simulink model "UNICO"  (R2023b)
settings: Solver=FixedStepDiscrete  StartTime=0.0  StopTime=inf  FixedStep=Control.DT  RelTol=1e-3
values from neighbouring files (symbols this model uses):
  Control =     [Parameters_UNICO.mat]
libraries: simulink x2
(part 1 of 3)
settings Model: Creator=evansolingen  LastModifiedBy=STUDENTE
settings SolverCC: AlgebraicLoopSolver=TrustRegion
settings DataIOCC: LimitDataPoints=on  SaveFormat=Array  SignalLoggingSaveFormat=ModelDataLogs  SaveOutput=off  SignalLogging=off  SaveTime=off  ReturnWorkspaceOutputs=off
settings OptimizationCC: BlockReduction=off  DefaultParameterBehavior=Inlined  BufferReuse=off  ReuseModelBlockBuffer=off  ExpressionDepthLimit=2147483647  LifeSpan=inf
settings DebuggingCC: UnderspecifiedInitializationDetection=Classic  MergeDetectMultiDrivingBlocksExec=none  SolverPrmCheckMsg=warning  MultiTaskDSMMsg=warning  MultiTaskCondExecSysMsg=none  FcnCallInpInsideContextMsg=warning  UnconnectedInputMsg=warning  UnconnectedOutputMsg=warning  UnconnectedLineMsg=warning  AllowSymbolicDim=off  StateNameClashWarn=warning  SFUnexpectedBacktrackingDiag=warning  SFNoUnconditionalDefaultTransitionDiag=warning  SFExecutionAtInitializationDiag=none  ArithmeticOperatorsInVariantConditions=warning
settings HardwareCC: ProdBitPerPointer=32  ProdBitPerSizeT=32  ProdBitPerPtrDiffT=32  ProdLargestAtomicFloat=None  ProdIntDivRoundTo=Undefined  ProdEndianess=Unspecified  ProdWordSize=32  ProdHWDeviceType=32-bit Generic
settings ModelReferenceCC: UpdateModelReferenceTargets=Force  EnableRefExpFcnMdlSchedulingChecks=on  PropagateSignalLabelsOutOfModel=off
settings SFSimCC: SimUseLocalCustomCode=off  SimParseCustomCode=off  CustomCodeUndefinedFunction=UseInterfaceOnly
settings RTWCC: Description=DISCON DLL Target (for use with GH BLADED)  SystemTargetFile=discon.tlc  TemplateMakefile=discon_vc.tmf  RTWUseLocalCustomCode=off
settings CodeAppCC: StateflowObjectComments=on
settings GRTTargetCC: TargetLangStandard=C89/C90 (ANSI)  CombineOutputUpdateFcns=off  GRTInterface=on  UseToolchainInfoCompliant=off  ExtModeMexFile=noextcomm
settings ConfigComp: CovMetricSettings=dw  CovSaveCumulativeToWorkspaceVar=on  CovSaveSingleToWorkspaceVar=on  CovExternalEMLEnable=off

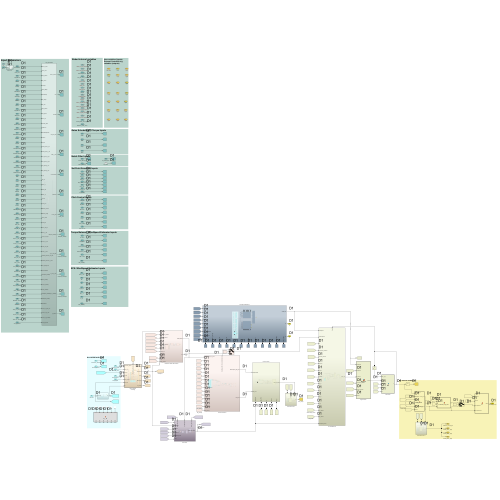
[thumbnail: Simulink's stored preview of the top-level diagram]
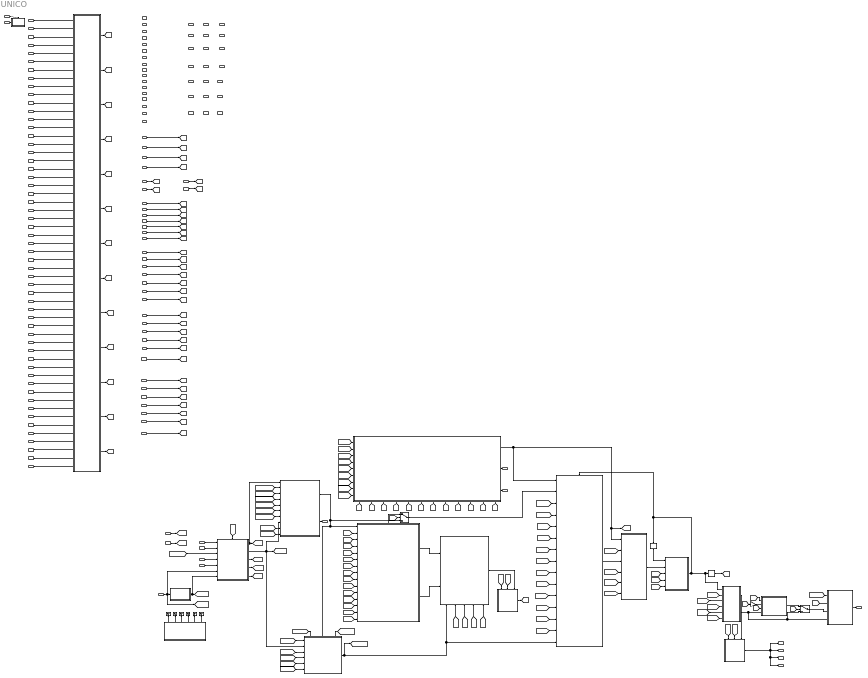
== system UNICO ==
  note: Bladed internal variables
  note: User variables (inputs)
      | External Controller log variables (outputs)
  note: Input parameters
  note: DLL OUTPUT INTERFACE
  note: DLL INTERFACE inputs
  note: Gains Scheduling PI Torque Inputs
  note: Torque Balance - WindSpeed Estimator Inputs
  note: Set Point Smoother Inputs
  note: EFK- WindSpeed Estimator Inputs
  note: Notch Filter Inputs
  note: Pitch Control Inputs
  Rated_Speed : Inport  PortDimensions=1
  Mode_Gain : Inport  Port=2  PortDimensions=1
  Blade1_OP_Root_Moment : Inport  Port=3  PortDimensions=1
  Blade2_OP_Root_Moment : Inport  Port=4  PortDimensions=1
  Blade3_OP_Root_Moment : Inport  Port=5  PortDimensions=1
  Rotor_Azimuth_Angle : Inport  Port=6  PortDimensions=1
  Init : Inport  Port=7  PortDimensions=1
  Shaft_Torque : Inport  Port=8  PortDimensions=1
  Blade1_IP_Root_Moment : Inport  Port=9  PortDimensions=1
  Blade2_IP_Root_Moment : Inport  Port=10  PortDimensions=1
  Blade3_IP_Root_Moment : Inport  Port=11  PortDimensions=1
  YawError : Inport  Port=12  PortDimensions=1
  YawBearingRate : Inport  Port=13  PortDimensions=1
  ElectricalPower : Inport  Port=14  PortDimensions=1
  Fore_Aft_Tower_Accel : Inport  Port=15  PortDimensions=1
  Generator_Speed : Inport  Port=16  PortDimensions=1
  Sidewards_Tower_Accel : Inport  Port=17  PortDimensions=1
  Below_Rated_Pitch_Angle : Inport  Port=18  PortDimensions=1
  Wind_Speed : Inport  Port=19  PortDimensions=1
  Com_dt : Inport  Port=20  PortDimensions=1
  SimTime : Inport  Port=21
  dKSwitch : Inport  Port=22  SampleTime=Control.DT  Interpolate=off  LockScale=on
  dRgn2K : Inport  Port=23  PortDimensions=1
  dOMSpdSwitch : Inport  Port=24  PortDimensions=1
  dRotorRadius : Inport  Port=25  PortDimensions=1
  dRgn3Mode : Inport  Port=26  PortDimensions=1
  dMRgn3Lin : Inport  Port=27  PortDimensions=1
  dGenEff : Inport  Port=28  PortDimensions=1
  dMinOMSpd : Inport  Port=29  PortDimensions=1
  dRtWSpd : Inport  Port=30  PortDimensions=1
  dRhoAir : Inport  Port=31  PortDimensions=1
  dRtPwr : Inport  Port=32  PortDimensions=1
  dRtGenSpd : Inport  Port=33  PortDimensions=1
  dTSRopt : Inport  Port=34  PortDimensions=1
  dRgn2Mode : Inport  Port=35  PortDimensions=1
  dWindSpeedFSw : Inport  Port=36
  dWindSpeedFLPF : Inport  Port=37
  dGenSpeedFSw : Inport  Port=38
  dGenSpeedFLPF : Inport  Port=39
  dRefSpeedFSw : Inport  Port=40
  dRefSpeedFLPF : Inport  Port=41
  dVLin : Inport  Port=42
  dMaxRat : Inport  Port=43  PortDimensions=1
  dMaxTq : Inport  Port=44  PortDimensions=1
  dMinTq : Inport  Port=45  PortDimensions=1
  dRtTq : Inport  Port=46  PortDimensions=1
  dEcho : Inport  Port=47
  dCpMax : Inport  Port=48
  dFPitch : Inport  Port=49
  Measured_Torque : Inport  Port=50
  dMinOMSpdSwitch : Inport  Port=51  PortDimensions=1
  Architecture_Selector : Inport  Port=52
  dZeros_Damping : Inport  Port=53
  dPoles_Damping : Inport  Port=54
  dBlades_Number : Inport  Port=55
  dBlades_Height : Inport  Port=56
  dAWSwitch : Inport  Port=57
  dKpBr : Inport  Port=58  PortDimensions=1
  dRotInertia : Inport  Port=59
  dIntTermSwitch : Inport  Port=60
  dKiBr : Inport  Port=61  PortDimensions=1
  dKpAr : Inport  Port=62  PortDimensions=1
  dKiAr : Inport  Port=63  PortDimensions=1
  dTSR_R3 : Inport  Port=64
  Measured_Pitch : Inport  Port=65  PortDimensions=1
  Pitch_LPF_Sw : Inport  Port=66
  Torque_in_LPF_Sw : Inport  Port=67
  Power_LPF_Sw : Inport  Port=68
  Pitch_F_LPF : Inport  Port=69
  Torque_in_F_LPF : Inport  Port=70
  Power_F_LPF : Inport  Port=71
  SPS_LPF_Sw : Inport  Port=72
  SPS_F_LPF : Inport  Port=73
  SPS_Mode : Inport  Port=74
  SPS_Kvs : Inport  Port=75
  SPS_Kpc : Inport  Port=76
  SPS_Abbas_Factor : Inport  Port=77
  Max_Pitch : Inport  Port=78
  Pitch_Rate : Inport  Port=79
  LPF_StartingTime : Inport  Port=80
  WSE_Mode : Inport  Port=81
  GearBox_Ratio : Inport  Port=82
  Darrieus_Selector : Inport  Port=83
  Rotor_Area : Inport  Port=84
  Process_Noise_Q : Inport  Port=85
  Measurement_Noise_R : Inport  Port=86
  TBE_F_LPF : Inport  Port=87
  EKF_F_LPF : Inport  Port=88
  Rm : Inport  Port=89
  Ti : Inport  Port=90
  PS_LPF_Sw : Inport  Port=91
  PS_F_LPF : Inport  Port=92
  Min_Pitch : Inport  Port=93
  PC_Kp : Inport  Port=94
  PC_Ki : Inport  Port=95
  Cp_interp : Inport  Port=96
  Cp_opt_in : Inport  Port=97
  Cp_2_in : Inport  Port=98
  A_op : Inport  Port=99
  WindSpeed_PreWarp : Inport  Port=100
  GenSpeed_PreWarp : Inport  Port=101
  RefSpeed_PreWarp : Inport  Port=102
  Pitch_PreWarp : Inport  Port=103
  Torque_in_PreWarp : Inport  Port=104
  TBE_PreWarp : Inport  Port=105
  EKF_PreWarp : Inport  Port=106
  Power_PreWarp : Inport  Port=107
  SPS_PreWarp : Inport  Port=108
  PS_PreWarp : Inport  Port=109
  Pitch_Ctrl_Sw : Inport  Port=110
  Torque_out_LPF_Sw : Inport  Port=111
  Torque_out_F_LPF : Inport  Port=112
  Torque_out_PreWarp : Inport  Port=113
  NF_StartingTime : Inport  Port=114
  NF_Switch : Inport  Port=115
  omega_stallmin : Inport  Port=116
  Delay One Step : Delay  DelayLength=1
  Delay One Step3 : Delay  DelayLength=1
  Echo print : Subsystem
      settings: PortSchema="{\"entries\":[{\"content\":{\"sides\":[{\"content\":{\"connectorIds\":[\"In1\"]},\"type\":\"ConnectorPlacement.EquallySpacedRectSide\",\"uuid\":\"a7404841-4279-4901-8e4b-4d9f651fd70d\"},{\"content\":{\"side\":\"RIGHT\"},\"type\":\"ConnectorPlacement.EquallySpacedRectSide\",\"uuid\":\"c083252d-994d-448b-85dd-b05fa098362a\"},{\"content\":{\"connectorIds\":[\"In2\"],\"side\":\"TOP\"},\"type\":\"ConnectorPlacement.EquallySpacedRectSide\",\"uuid\":\"2158789e-5709-45dd-87ec-c3c83921db3a\"}]},\"type\":\"ConnectorPlacement.EquallySpacedConnector\",\"uuid\":\"2f3f8f4d-3210-4d41-988d-02cc8661526f\"}],\"packageUris\":[\"http://schema.mathworks.com/mf0/Connector/R2020b\"],\"version\":\"1.0\"}"
  Extract Signals & Filtering : Subsystem  TreatAsAtomicUnit=on
      settings: PortSchema="{\"entries\":[{\"content\":{\"sides\":[{\"content\":{\"connectorIds\":[\"In1\",\"In2\",\"In3\",\"In4\",\"In5\",\"In6\",\"In7\"]},\"type\":\"ConnectorPlacement.EquallySpacedRectSide\",\"uuid\":\"a404705e-4872-4bcb-ba41-9c444b954adf\"},{\"content\":{\"connectorIds\":[\"Out1\",\"Out2\",\"Out3\",\"Out4\",\"Out5\"],\"side\":\"RIGHT\"},\"type\":\"ConnectorPlacement.EquallySpacedRectSide\",\"uuid\":\"c545baa2-32cf-46ec-85e6-24376232facc\"},{\"content\":{\"connectorIds\":[\"In8\"],\"side\":\"TOP\"},\"type\":\"ConnectorPlacement.EquallySpacedRectSide\",\"uuid\":\"109e9702-ec3d-43ff-9af6-4bdbb05ed40a\"}]},\"type\":\"ConnectorPlacement.EquallySpacedConnector\",\"uuid\":\"3e4fa54c-da00-45a5-8912-ad9d54069fc2\"}],\"packageUris\":[\"http://schema.mathworks.com/mf0/Connector/R2020b\"],\"version\":\"1.0\"}"
  Gain4 : Gain  Gain=2*pi
  Input_parameters : Subsystem
  MATLAB Function1 : MATLAB Function  TreatAsAtomicUnit=on
  MATLAB Function2 : MATLAB Function  TreatAsAtomicUnit=on
  MATLAB Function3 : MATLAB Function  TreatAsAtomicUnit=on
  MATLAB Function4 : MATLAB Function  TreatAsAtomicUnit=on
  Notch Filter : Subsystem
      settings: PortSchema="{\"entries\":[{\"content\":{\"sides\":[{\"content\":{\"connectorIds\":[\"In1\",\"In2\",\"In3\",\"In4\",\"In5\",\"In6\"]},\"type\":\"ConnectorPlacement.EquallySpacedRectSide\",\"uuid\":\"266d7f1f-a9f2-4128-b770-569d38332992\"},{\"content\":{\"connectorIds\":[\"Out1\"],\"side\":\"RIGHT\"},\"type\":\"ConnectorPlacement.EquallySpacedRectSide\",\"uuid\":\"006e736b-d915-4b42-8363-b4fafec53ea5\"},{\"content\":{\"connectorIds\":[\"In7\",\"In8\",\"In9\"],\"side\":\"TOP\"},\"type\":\"ConnectorPlacement.EquallySpacedRectSide\",\"uuid\":\"979f8782-bd32-4411-8fc6-7070b3b90e64\"},{\"content\":{\"side\":\"BOTTOM\"},\"type\":\"ConnectorPlacement.EquallySpacedRectSide\",\"uuid\":\"d10cf628-97fc-4eef-9b08-34d81c8bbc38\"}]},\"type\":\"ConnectorPlacement.EquallySpacedConnector\",\"uuid\":\"1a915c26-6e95-4b6d-8a27-3bc1b56b8115\"}],\"packageUris\":[\"http://schema.mathworks.com/mf0/Connector/R2020b\"],\"version\":\"1.0\"}"
  PI CONTROLLER : Subsystem
      settings: PortSchema="{\"entries\":[{\"content\":{\"sides\":[{\"content\":{\"connectorIds\":[\"In1\",\"In2\",\"In3\",\"In4\",\"In5\",\"In6\",\"In7\",\"In8\",\"In9\",\"In10\",\"In11\",\"In12\",\"In13\",\"In14\",\"In15\"]},\"type\":\"ConnectorPlacement.EquallySpacedRectSide\",\"uuid\":\"cac6f54d-e2c8-43c6-b064-9a31ea99ed9a\"},{\"content\":{\"connectorIds\":[\"Out1\"],\"side\":\"RIGHT\"},\"type\":\"ConnectorPlacement.EquallySpacedRectSide\",\"uuid\":\"e149802a-12fb-4560-9018-b92a983da9c3\"},{\"content\":{\"connectorIds\":[\"In16\"],\"side\":\"TOP\"},\"type\":\"ConnectorPlacement.EquallySpacedRectSide\",\"uuid\":\"c9e2d139-52ab-4592-996b-9b011a50426a\"}]},\"type\":\"ConnectorPlacement.EquallySpacedConnector\",\"uuid\":\"845cf794-e810-4ec5-9bce-289872a07b1e\"}],\"packageUris\":[\"http://schema.mathworks.com/mf0/Connector/R2020b\"],\"version\":\"1.0\"}"
  Pitch Controller : Subsystem
      settings: PortSchema="{\"entries\":[{\"content\":{\"sides\":[{\"content\":{\"connectorIds\":[\"In1\",\"In2\"]},\"type\":\"ConnectorPlacement.EquallySpacedRectSide\",\"uuid\":\"15f3ef00-8fd2-4b01-b950-6d151530d8d8\"},{\"content\":{\"connectorIds\":[\"Out1\"],\"side\":\"RIGHT\"},\"type\":\"ConnectorPlacement.EquallySpacedRectSide\",\"uuid\":\"9a379538-e873-4d9a-b3d5-9d5b8b382616\"},{\"content\":{\"side\":\"TOP\"},\"type\":\"ConnectorPlacement.EquallySpacedRectSide\",\"uuid\":\"382e266d-b53f-4a4d-a6cd-b7a4030212ef\"},{\"content\":{\"connectorIds\":[\"In3\",\"In4\",\"In5\",\"In6\",\"In7\"],\"side\":\"BOTTOM\"},\"type\":\"ConnectorPlacement.EquallySpacedRectSide\",\"uuid\":\"ee17fbc2-2aec-488d-9e0d-2e4dec5ded05\"}]},\"type\":\"ConnectorPlacement.EquallySpacedConnector\",\"uuid\":\"dba4a2db-8eaa-452b-8e55-416d9caf5878\"}],\"packageUris\":[\"http://schema.mathworks.com/mf0/Connector/R2020b\"],\"version\":\"1.0\"}"
  Pitch Rate Limiter : Subsystem
      settings: PortSchema="{\"entries\":[{\"content\":{\"sides\":[{\"content\":{\"connectorIds\":[\"In1\",\"In2\",\"In3\"]},\"type\":\"ConnectorPlacement.EquallySpacedRectSide\",\"uuid\":\"71de1963-385a-424e-a4e7-bb08b9d03775\"},{\"content\":{\"side\":\"RIGHT\"},\"type\":\"ConnectorPlacement.EquallySpacedRectSide\",\"uuid\":\"e3763a80-b3da-4c7c-ac2e-798dc78d2a39\"},{\"content\":{\"side\":\"TOP\"},\"type\":\"ConnectorPlacement.EquallySpacedRectSide\",\"uuid\":\"c338073c-3d17-477d-80b8-b5d5ee58aec7\"},{\"content\":{\"connectorIds\":[\"Out1\"],\"side\":\"BOTTOM\"},\"type\":\"ConnectorPlacement.EquallySpacedRectSide\",\"uuid\":\"70822ac6-7ea9-4832-9fee-c86b7b7e7f31\"}]},\"type\":\"ConnectorPlacement.EquallySpacedConnector\",\"uuid\":\"46c33881-c4d8-4782-931d-07fcd796c079\"}],\"packageUris\":[\"http://schema.mathworks.com/mf0/Connector/R2020b\"],\"version\":\"1.0\"}"
  Pitch Rate Limiter1 : Subsystem
      settings: PortSchema="{\"entries\":[{\"content\":{\"sides\":[{\"content\":{\"connectorIds\":[\"In1\",\"In2\",\"In3\"]},\"type\":\"ConnectorPlacement.EquallySpacedRectSide\",\"uuid\":\"71de1963-385a-424e-a4e7-bb08b9d03775\"},{\"content\":{\"side\":\"RIGHT\"},\"type\":\"ConnectorPlacement.EquallySpacedRectSide\",\"uuid\":\"e3763a80-b3da-4c7c-ac2e-798dc78d2a39\"},{\"content\":{\"side\":\"TOP\"},\"type\":\"ConnectorPlacement.EquallySpacedRectSide\",\"uuid\":\"c338073c-3d17-477d-80b8-b5d5ee58aec7\"},{\"content\":{\"connectorIds\":[\"Out1\"],\"side\":\"BOTTOM\"},\"type\":\"ConnectorPlacement.EquallySpacedRectSide\",\"uuid\":\"70822ac6-7ea9-4832-9fee-c86b7b7e7f31\"}]},\"type\":\"ConnectorPlacement.EquallySpacedConnector\",\"uuid\":\"46c33881-c4d8-4782-931d-07fcd796c079\"}],\"packageUris\":[\"http://schema.mathworks.com/mf0/Connector/R2020b\"],\"version\":\"1.0\"}"
  Rate limiter : MATLAB Function  TreatAsAtomicUnit=on
  Reference Speed Determination : Subsystem
  "Region Switch " : MATLAB Function  TreatAsAtomicUnit=on
  Set Point Smoother : Subsystem
      settings: PortSchema="{\"entries\":[{\"content\":{\"sides\":[{\"content\":{\"connectorIds\":[\"In1\",\"In2\",\"In3\",\"In4\",\"In5\",\"In6\",\"In7\",\"In8\",\"In9\",\"In10\",\"In11\",\"In12\",\"In13\",\"In14\",\"In15\"]},\"type\":\"ConnectorPlacement.EquallySpacedRectSide\",\"uuid\":\"b45f5cc4-c36d-4f69-abed-54c577fa7509\"},{\"content\":{\"connectorIds\":[\"Out1\",\"Out2\"],\"side\":\"RIGHT\"},\"type\":\"ConnectorPlacement.EquallySpacedRectSide\",\"uuid\":\"93d4c31e-6d03-43b5-9766-df680cc2625e\"},{\"content\":{\"connectorIds\":[\"Out3\"],\"side\":\"TOP\"},\"type\":\"ConnectorPlacement.EquallySpacedRectSide\",\"uuid\":\"bbab9ad3-67d7-4805-8de6-8e5f911d7e32\"}]},\"type\":\"ConnectorPlacement.EquallySpacedConnector\",\"uuid\":\"cc63daf0-1a6c-427a-a186-92445beec46e\"}],\"packageUris\":[\"http://schema.mathworks.com/mf0/Connector/R2020b\"],\"version\":\"1.0\"}"
  Subsystem1 : Subsystem
  Switch : Switch  Criteria=u2 ~= 0  SaturateOnIntegerOverflow=off  InputSameDT=off
  Switch3 : Switch  Criteria=u2 ~= 0  SaturateOnIntegerOverflow=off  InputSameDT=off
  Terminator{1..6} (6 alike) : Terminator
  Wind Speed Estimators : Subsystem
      settings: PortSchema="{\"entries\":[{\"content\":{\"sides\":[{\"content\":{\"connectorIds\":[\"In1\",\"In2\",\"In3\",\"In4\",\"In5\",\"In6\",\"In7\",\"In8\",\"In9\"]},\"type\":\"ConnectorPlacement.EquallySpacedRectSide\",\"uuid\":\"93f714cb-9c59-4e12-ade1-e7df00512455\"},{\"content\":{\"connectorIds\":[\"Out1\",\"Out2\",\"Out3\"],\"side\":\"RIGHT\"},\"type\":\"ConnectorPlacement.EquallySpacedRectSide\",\"uuid\":\"d5526135-9f63-41d7-93a5-f87b80e4f455\"},{\"content\":{\"side\":\"TOP\"},\"type\":\"ConnectorPlacement.EquallySpacedRectSide\",\"uuid\":\"82fe9337-8013-44e5-aac2-a73e686a79d7\"},{\"content\":{\"connectorIds\":[\"In10\",\"In11\",\"In12\",\"In13\",\"In14\",\"In15\",\"In16\",\"In17\",\"In18\",\"In19\",\"In20\",\"In21\"],\"side\":\"BOTTOM\"},\"type\":\"ConnectorPlacement.EquallySpacedRectSide\",\"uuid\":\"b65e2683-3e9b-43b5-8446-61ba0d8b1898\"}]},\"type\":\"ConnectorPlacement.EquallySpacedConnector\",\"uuid\":\"740892b4-794b-4135-9713-ff5336da8300\"}],\"packageUris\":[\"http://schema.mathworks.com/mf0/Connector/R2020b\"],\"version\":\"1.0\"}"
  Log3 : Outport  PortDimensions=1  VectorParamsAs1DForOutWhenUnconnected=off
  Log4 : Outport  Port=2  PortDimensions=1  VectorParamsAs1DForOutWhenUnconnected=off
  Log5 : Outport  Port=3  PortDimensions=1  VectorParamsAs1DForOutWhenUnconnected=off
  Log6 : Outport  Port=4  PortDimensions=1  VectorParamsAs1DForOutWhenUnconnected=off
  Log7 : Outport  Port=5  PortDimensions=1  VectorParamsAs1DForOutWhenUnconnected=off
  Log10 : Outport  Port=6  PortDimensions=1  VectorParamsAs1DForOutWhenUnconnected=off
  Log8 : Outport  Port=7  PortDimensions=1  VectorParamsAs1DForOutWhenUnconnected=off
  Log20 : Outport  Port=8  PortDimensions=1  VectorParamsAs1DForOutWhenUnconnected=off
  Log12 : Outport  Port=9  PortDimensions=1  VectorParamsAs1DForOutWhenUnconnected=off
  Log17 : Outport  Port=10  PortDimensions=1  VectorParamsAs1DForOutWhenUnconnected=off
  Log18 : Outport  Port=11  PortDimensions=1  VectorParamsAs1DForOutWhenUnconnected=off
  Log19 : Outport  Port=12  PortDimensions=1  VectorParamsAs1DForOutWhenUnconnected=off
  Log13 : Outport  Port=13  PortDimensions=1  VectorParamsAs1DForOutWhenUnconnected=off
  Log14 : Outport  Port=14  PortDimensions=1  VectorParamsAs1DForOutWhenUnconnected=off
  Log15 : Outport  Port=15  PortDimensions=1  VectorParamsAs1DForOutWhenUnconnected=off
  Log1 : Outport  Port=16  PortDimensions=1  VectorParamsAs1DForOutWhenUnconnected=off
  Log16 : Outport  Port=17  PortDimensions=1  VectorParamsAs1DForOutWhenUnconnected=off
  Log2 : Outport  Port=18  PortDimensions=1  VectorParamsAs1DForOutWhenUnconnected=off
  Log9 : Outport  Port=19  PortDimensions=1  VectorParamsAs1DForOutWhenUnconnected=off
  Log11 : Outport  Port=20  PortDimensions=1  VectorParamsAs1DForOutWhenUnconnected=off
  Yaw_Rate : Outport  Port=21  PortDimensions=1  VectorParamsAs1DForOutWhenUnconnected=off
  Blade1_Pitch_Angle : Outport  Port=22  PortDimensions=1  VectorParamsAs1DForOutWhenUnconnected=off
  Blade2_Pitch_Angle : Outport  Port=23  PortDimensions=1  VectorParamsAs1DForOutWhenUnconnected=off
  Blade3_Pitch_Angle : Outport  Port=24  PortDimensions=1  VectorParamsAs1DForOutWhenUnconnected=off
  Collective_Pitch_Angle : Outport  Port=25  PortDimensions=1  VectorParamsAs1DForOutWhenUnconnected=off
  vh : Outport  Port=26
  vw : Outport  Port=27
  Generator_Torque : Outport  Port=28  PortDimensions=1  VectorParamsAs1DForOutWhenUnconnected=off
  Cp : Outport  Port=29
  tag scope: InPar=global, KiAr=global, KiBr=global, KpAr=global, KpBr=global, LPF=global, MaxRat=global, SPS_F_LPF=global, SPS_F_Sw=global
  wires:
  dRhoAir/1 -> Input_parameters/4(dAir_Dens)
  dMaxRat/1 -> Input_parameters/27(dMax_Rat)
  dRgn2K/1 -> Input_parameters/17(Rgn2K)
  Init/1 -> Echo print/1(Init)
  dKSwitch/1 -> Input_parameters/16(KSwitch)
  dFPitch/1 -> Input_parameters/30(fixed_pitch)
  dTSRopt/1 -> Input_parameters/5(dTSRopt)
  Input_parameters/2(LPF) -> [LPF]
  dWindSpeedFLPF/1 -> Input_parameters/19(Wind_Speed_F_LPF)
  dRgn2Mode/1 -> Input_parameters/3(dRgn2_Mode)
  Input_parameters/1(Discon_Params) -> [InPar]
  dEcho/1 -> Echo print/2(Echo)
  dRefSpeedFLPF/1 -> Input_parameters/23(Ref_Speed_F_LPF)
  dRtTq/1 -> Input_parameters/25(dRt_Tq)
  dVLin/1 -> Input_parameters/24(V_lin)
  dRefSpeedFSw/1 -> Input_parameters/22(Ref_Speed_F_Sw)
  dRtGenSpd/1 -> Input_parameters/7(dRatGenSpd)
  dMaxTq/1 -> Input_parameters/28(dMax_Tq)
  dOMSpdSwitch/1 -> Input_parameters/14(SpdSwitch)
  dRgn3Mode/1 -> Input_parameters/10(dRgn3_Mode)
  dCpMax/1 -> Input_parameters/29(Cpmax)
  dRotorRadius/1 -> Input_parameters/1(dRotor_radius)
  dRtWSpd/1 -> Input_parameters/8(dRt_WSpd)
  dMinTq/1 -> Input_parameters/26(dMin_Tq)
  dMinOMSpd/1 -> Input_parameters/6(dMin_OMSpd)
  dMRgn3Lin/1 -> Input_parameters/11(dM_Rgn3Lin)
  dRtPwr/1 -> Input_parameters/9(dRt_Pwr)
  dGenEff/1 -> Input_parameters/12(dGen_Eff)
  dGenSpeedFLPF/1 -> Input_parameters/21(Gen_Speed_F_LPF)
  dGenSpeedFSw/1 -> Input_parameters/20(Gen_Speed_F_Sw)
  dWindSpeedFSw/1 -> Input_parameters/18(Wind_Speed_F_Sw)
  dMinOMSpdSwitch/1 -> Input_parameters/15(dMinOMSpdSwitch)
  Input_parameters/3(MaxRat) -> [MaxRat]
  SimTime/1 -> Extract Signals & Filtering/6(SimTime), [simTime], Subsystem1/1(SimTime)
  Subsystem1/1(dt) -> Extract Signals & Filtering/7(dt), [dt]
  dZeros_Damping/1 -> [dZeros_Damping]
  dPoles_Damping/1 -> [dPoles_Damping]
  dBlades_Number/1 -> Input_parameters/31(dBlades_Number)
  "Region Switch "/1(GenTq) -> Rate limiter/2(Gen_Tq)
  [MaxRat] -> Rate limiter/3(dMaxRate)
  [InPar] -> "Region Switch "/6(Params)
  [simTime] -> Rate limiter/4(time)
  [InPar] -> Reference Speed Determination/4(InPar)
  Delay One Step3/1 -> Rate limiter/1(Gen_Tq_b)
  [dt] -> Rate limiter/5(dt)
  Architecture_Selector/1 -> [Architecture_Selector]
  [Architecture_Selector] -> "Region Switch "/4(Architecture_Selector)
  dBlades_Height/1 -> Input_parameters/32(dBlades_Height)
  Extract Signals & Filtering/2(GenSpeed) -> [Genspeed], Reference Speed Determination/8(GenSpeed), Notch Filter/2(GenSpeed)  "wg"
  Notch Filter/1(GenSpeed_filtered) -> [GenSpeed_Filtered], Pitch Controller/3(GenSpeed), PI CONTROLLER/15(GenSpeed_filtered)  "GenSpeed_filtered"
  [dt] -> Notch Filter/1(dt)
  [dZeros_Damping] -> Notch Filter/7(dZeros_Damping)
  [InPar] -> Notch Filter/6(InPar)
  [dPoles_Damping] -> Notch Filter/9(dPoles_Damping)
  [simTime] -> Notch Filter/3(SimTime)
  Reference Speed Determination/1(GenSpeedRef) -> Switch/3, Set Point Smoother/1(GenSpeed_Ref_Tq_contr), Notch Filter/8(DESGenSpeed)
  [Architecture_Selector] -> Reference Speed Determination/2(Architecture_Selector)
  [dt] -> PI CONTROLLER/3(dt)
  [Architecture_Selector] -> PI CONTROLLER/4(Architecture_Selector)
  [simTime] -> PI CONTROLLER/6(Simtime)
  [LimInt] -> PI CONTROLLER/7(LimInt)
  [InPar] -> PI CONTROLLER/8(Params)
  [KpAr] -> PI CONTROLLER/9(kp_ar)
  [KiAr] -> PI CONTROLLER/10(ki_ar)
  [KpBr] -> PI CONTROLLER/11(kp_br)
  [KiBr] -> PI CONTROLLER/12(ki_br)
  PI CONTROLLER/1(Gen_Tq) -> "Region Switch "/3(PI_GenTq)
  [GenSpeed_Filtered] -> "Region Switch "/2(GenSpeed)
  [dIntTermSat_Switch] -> PI CONTROLLER/13(ITS_Switch)
  dRotInertia/1 -> Input_parameters/33(Rotor_Inertia)
  [dAWSwitch] -> PI CONTROLLER/14(AW_Switch)
  dKpBr/1 -> [KpBr]
  dTSR_R3/1 -> Input_parameters/34(dTSR_R3)
  dKpAr/1 -> [KpAr]
  dKiAr/1 -> [KiAr]
  Pitch Controller/1(Pitch_out (rad)) -> Pitch Rate Limiter/3(pitch [rad])
  [dt] -> Pitch Controller/5(dt)
  Pitch Rate Limiter/1(s) -> [Pitch_Output]
  [InPar] -> Set Point Smoother/10(In_Params)
  Delay One Step/1 -> [Gen_Torque]
  [dt] -> Pitch Rate Limiter/1(dt)
  Set Point Smoother/1(RatGenSpeed_Ref_pitch) -> Pitch Controller/1(GenSpeedRef)
  [Power] -> Set Point Smoother/5(Power)
  [Pitch] -> Set Point Smoother/6(Pitch)
  Extract Signals & Filtering/5(El_Power) -> [Power]
  Extract Signals & Filtering/3(Pitch) -> [Pitch]
  Wind_Speed/1 -> Extract Signals & Filtering/5(Wind_speed)
  ElectricalPower/1 -> Extract Signals & Filtering/4(Power)
  [Gen_Torque] -> Extract Signals & Filtering/3(Torque)
  Measured_Pitch/1 -> Extract Signals & Filtering/2(Pitch_in)
  [LPF] -> Extract Signals & Filtering/8(Wind_Filter_Parameters)
  Extract Signals & Filtering/1(WindSpeed) -> [WindSpeed], Reference Speed Determination/1(WindSpeed)
  Extract Signals & Filtering/4(GenTorque) -> [GenTorque]
  Switch/1 -> PI CONTROLLER/2(DesGenSpeed)
  Pitch_LPF_Sw/1 -> Input_parameters/35(Pitch_LPF_Sw)
  Pitch_F_LPF/1 -> Input_parameters/36(Pitch_F_LPF)
  Torque_in_LPF_Sw/1 -> Input_parameters/37(Torque_LPF_Sw)
  Torque_in_F_LPF/1 -> Input_parameters/38(Torque_F_LPF)
  Power_LPF_Sw/1 -> Input_parameters/39(Power_LPF_Sw)
  Power_F_LPF/1 -> Input_parameters/40(Power_F_LPF)
  SPS_LPF_Sw/1 -> Input_parameters/41(SetPoint_Smoother_LPF_Sw)
  SPS_F_LPF/1 -> Input_parameters/42(SetPoint_Smoother_F_LPF)
  SPS_Mode/1 -> [SetPoint_Smoother_Mode]
  SPS_Kvs/1 -> [Kvs]
  SPS_Kpc/1 -> [Kpc]
  [Kpc] -> Set Point Smoother/8(Kpc)
  [Kvs] -> Set Point Smoother/7(Kvs)
  SPS_Abbas_Factor/1 -> [Abbas_Factor]
  [Abbas_Factor] -> Set Point Smoother/9(Abbas_NormFactor)
  Input_parameters/5(SPS_F_LPF) -> [SPS_F_LPF]
  [SPS_F_Sw] -> Set Point Smoother/12(SPS_LPF_Sw)
  [SPS_F_LPF] -> Set Point Smoother/11(SPS_F_LPF)
  Pitch_Rate/1 -> [Pitch_Rate]
  Max_Pitch/1 -> [Max_Pitch]
  Set Point Smoother/2(Min_Pitch) -> Pitch Controller/2(Min_Pitch)
  [Max_Pitch] -> Pitch Controller/4(Max_Pitch)
  [Pitch_Rate] -> Pitch Rate Limiter/2(Pitch_Rate)
  LPF_StartingTime/1 -> Input_parameters/43(LPF_StartingTime)
  [WindSpeed] -> Wind Speed Estimators/6(WSpeed)
  [dt] -> Wind Speed Estimators/3(dt)
  [simTime] -> Wind Speed Estimators/2(time)
  [Genspeed] -> Wind Speed Estimators/4(GenSpeed)
  [GenTorque] -> Wind Speed Estimators/5(GenTorque)
  WSE_Mode/1 -> [WSE_Mode]
  [WSE_Mode] -> Wind Speed Estimators/9(WSE_Mode)
  GearBox_Ratio/1 -> Input_parameters/13(GearBox_Ratio)
  [InPar] -> Wind Speed Estimators/1(InParameters)
  [Architecture_Selector] -> Wind Speed Estimators/7(Architecture_Selector)
  Darrieus_Selector/1 -> [Darrieus_Selector]
  Rotor_Area/1 -> Input_parameters/2(Rotor_Area)
  [Darrieus_Selector] -> Reference Speed Determination/3(Darrieus_Selector)
  [Darrieus_Selector] -> Wind Speed Estimators/8(Darrieus_Selector)
  [Darrieus_Selector] -> PI CONTROLLER/5(Darrieus_Selector)
  [Darrieus_Selector] -> "Region Switch "/5(Darrieus_Selector)
  TBE_F_LPF/1 -> [TBE_L_LPF]
  Measurement_Noise_R/1 -> [R]
  Process_Noise_Q/1 -> [Q]
  [TBE_L_LPF] -> Wind Speed Estimators/12(TBE_F_LPF)
  [R] -> Wind Speed Estimators/11(Measurement_Noise_R)
  [Q] -> Wind Speed Estimators/10(Process_Noise_Q)
  EKF_F_LPF/1 -> [EKF_L_LPF]
  [EKF_L_LPF] -> Wind Speed Estimators/13(EKF_F_LPF)
  Rm/1 -> [MN_Covariance]
  [MN_Covariance] -> Wind Speed Estimators/14(Rm)
  [Ti] -> Wind Speed Estimators/15(Ti)
  PS_F_LPF/1 -> [PS_F_LPF]
  PS_LPF_Sw/1 -> [PS_LPF_Sw]
  [PS_LPF_Sw] -> Set Point Smoother/3(PS_LPF_Sw)
  [PS_F_LPF] -> Set Point Smoother/4(PS_F_LPF)
  Input_parameters/4(SPS_LPF_Sw) -> [SPS_F_Sw]
  Set Point Smoother/3(GenSpeed_Ref_Tq_Controller_Smoothed) -> Switch/1
  [SetPoint_Smoother_Mode] -> Switch/2
  [pitch_min] -> Set Point Smoother/13(pitch_min)
  Min_Pitch/1 -> [pitch_min]
  PC_Ki/1 -> [PC_Ki]
  PC_Kp/1 -> [PC_Kp]
  [PC_Kp] -> Pitch Controller/6(PC_Kp)
  [PC_Ki] -> Pitch Controller/7(PC_Ki)
  [Cp_interp] -> Wind Speed Estimators/16(Cp_interp)
  Cp_interp/1 -> [Cp_interp]
  [Cp_opt_in] -> Wind Speed Estimators/17(Cp_opt_in)
  [Cp_2_in] -> Wind Speed Estimators/18(Cp_2_in)
  [A_op] -> Wind Speed Estimators/19(A_op)
  Cp_opt_in/1 -> [Cp_opt_in]
  Cp_2_in/1 -> [Cp_2_in]
  A_op/1 -> [A_op]
  Wind Speed Estimators/3(vw) -> vw/1
  Wind Speed Estimators/2(vh) -> vh/1
  Generator_Speed/1 -> Extract Signals & Filtering/1(Generator_speed)
  Ti/1 -> [Ti]
  dKiBr/1 -> [KiBr]
  Input_parameters/6(IntTermSwitch) -> [dIntTermSat_Switch]
  Input_parameters/7(AWSwitch) -> [dAWSwitch]
  dIntTermSwitch/1 -> Input_parameters/44(dIntTermSwitch)
  Input_parameters/8(Fixed_pitch) -> [Fxd_Pitch]
  MATLAB Function1/1(Pitch_out) -> Pitch Rate Limiter1/3(pitch [rad])
  [Pitch_Output] -> MATLAB Function1/5(Pitch_Controller_Out)
  [dt] -> Reference Speed Determination/6(dt)
  [dt] -> Set Point Smoother/2(dt)
  GenSpeed_PreWarp/1 -> Input_parameters/45(GenSpeed_PreWarp)
  Pitch_PreWarp/1 -> Input_parameters/46(Pitch_PreWarp)
  Torque_in_PreWarp/1 -> Input_parameters/47(Torque_PreWarp)
  dAWSwitch/1 -> Input_parameters/51(dAWSwitch)
  EKF_PreWarp/1 -> [EKF_PreWarp]
  TBE_PreWarp/1 -> [TBE_PreWarp]
  Power_PreWarp/1 -> Input_parameters/48(Power_PreWarp)
  SPS_PreWarp/1 -> [SPS_PreWarp]
  PS_PreWarp/1 -> [PS_PreWarp]
  WindSpeed_PreWarp/1 -> Input_parameters/49(WindSpeed_PreWarp)
  RefSpeed_PreWarp/1 -> Input_parameters/50(RefSpeed_PreWarp)
  Input_parameters/9(Refspeed_PreWarp) -> [RefSpeed_PreWarp]
  [RefSpeed_PreWarp] -> Reference Speed Determination/5(RefSpeed_PreWarp)
  [SPS_PreWarp] -> Set Point Smoother/14(SPS_Prewarp)
  [PS_PreWarp] -> Set Point Smoother/15(PS_prewarp)
  [TBE_PreWarp] -> Wind Speed Estimators/20(TBE_PreWarp)
  [EKF_PreWarp] -> Wind Speed Estimators/21(EKF_PreWarp)
  [Pitch_Ctrl_Sw] -> MATLAB Function1/4(Pitch_Ctrl_Sw)
  [InPar] -> MATLAB Function1/6(params)
  Pitch_Ctrl_Sw/1 -> [Pitch_Ctrl_Sw]
  [simTime] -> Reference Speed Determination/9(SimTime)
  [LPF] -> Reference Speed Determination/10(LPF_params)
  [Tq_out_LPF_Sw] -> Switch3/2
  MATLAB Function3/1(y) -> Switch3/1
  Gain4/1 -> MATLAB Function3/2(freq)
  [Tq_out_F_LPF] -> Gain4/1
  [Tq_out_PreWarp] -> MATLAB Function3/1(w0)
  [dt] -> MATLAB Function3/3(Ts)
  Torque_out_LPF_Sw/1 -> Input_parameters/52(Torque_out_LPF_Sw)
  Torque_out_F_LPF/1 -> Input_parameters/53(Torque_out_F_LPF)
  Torque_out_PreWarp/1 -> Input_parameters/54(Torque_out_PreWarp)
  Input_parameters/10(Tq_out_LPF_Sw) -> [Tq_out_LPF_Sw]
  Input_parameters/11(Tq_out_F_LPF) -> [Tq_out_F_LPF]
  Input_parameters/12(Tq_out_PreWarp) -> [Tq_out_PreWarp]
  Switch3/1 -> MATLAB Function4/3(GenTqFiltered)
  MATLAB Function1/2(Torque_out) -> MATLAB Function4/4(GenTqUnfiltered), Switch3/3, MATLAB Function3/4(u)
  [LPF] -> MATLAB Function4/2(params)
  [simTime] -> MATLAB Function4/1(SimTime)
  NF_StartingTime/1 -> [NF_Starting_Time]
  [NF_Starting_Time] -> Notch Filter/5(NF_StartingTime)
  NF_Switch/1 -> [NF_Switch]
  [NF_Switch] -> Notch Filter/4(NF_Switch)
  Reference Speed Determination/2(Cp) -> Cp/1
  omega_stallmin/1 -> Input_parameters/55(omega_stallmin)
  Input_parameters/13(w_stallmin) -> [wstallmin]
  [wstallmin] -> Reference Speed Determination/7(wstall_min)
  Rate limiter/1(s) -> MATLAB Function1/1(Torque_PI_out), Delay One Step/1, Delay One Step3/1, PI CONTROLLER/16(Sat_Tq)
  MATLAB Function4/1(GenTq) -> Generator_Torque/1
  MATLAB Function2/1(y1) -> Terminator1/1
  MATLAB Function2/2(y2) -> Terminator2/1
  MATLAB Function2/3(y3) -> Terminator3/1
  [dt] -> Pitch Rate Limiter1/1(dt)
  [Pitch_Rate] -> Pitch Rate Limiter1/2(Pitch_Rate)
  Wind Speed Estimators/1(WindSpeed) -> PI CONTROLLER/1(WindSpeed), "Region Switch "/1(WindSpeed), [Wind_Speed]
  [Wind_Speed] -> MATLAB Function1/2(WindSpeed)
  [Fxd_Pitch] -> MATLAB Function1/3(dFPitch)
  Pitch Rate Limiter1/1(s) -> Blade3_Pitch_Angle/1, Blade2_Pitch_Angle/1, Blade1_Pitch_Angle/1, Collective_Pitch_Angle/1
  MATLAB Function2/4(y4) -> Terminator4/1
  MATLAB Function2/5(y5) -> Terminator5/1
  MATLAB Function2/6(y6) -> Terminator6/1

== system UNICO/Echo print ==
  Init : Inport
  Echo : Inport  Port=2
  Enabled Subsystem : Subsystem  TreatAsAtomicUnit=on
      settings: LibrarySourceBlock=|
      | hdlsllib/Ports &
      | Subsystems/Enabled
      | Subsystem
  wires:
  [InPar] -> Enabled Subsystem/2(Params)
  [KpAr] -> Enabled Subsystem/3(KpAr)
  [KiAr] -> Enabled Subsystem/4(KiAr)
  [MaxRat] -> Enabled Subsystem/7(Max_Rat)
  Init/1 -> Enabled Subsystem/1(Init)
  [LPF] -> Enabled Subsystem/8(Params_WS_F)
  Echo/1 -> Enabled Subsystem/Enable
  [KpBr] -> Enabled Subsystem/5(KpBr)
  [KiBr] -> Enabled Subsystem/6(KiBr)

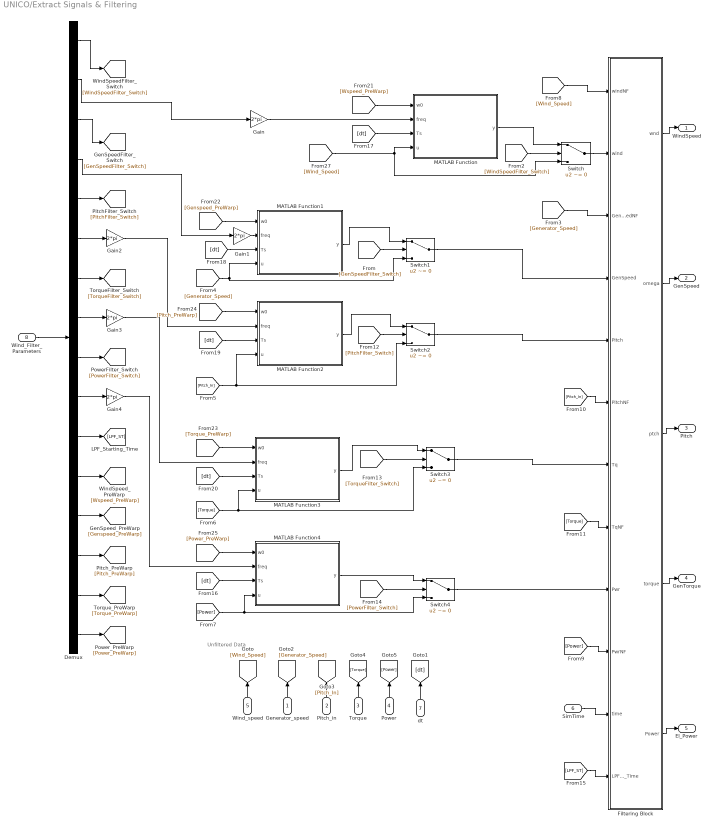
== system UNICO/Extract Signals & Filtering ==
  note: Unfiltered Data
  Generator_speed : Inport
  Pitch_in : Inport  Port=2
  Torque : Inport  Port=3
  Power : Inport  Port=4
  Wind_speed : Inport  Port=5
  SimTime : Inport  Port=6
  dt : Inport  Port=7
  Wind_Filter_Parameters : Inport  Port=8
  Demux : Demux  Outputs=16
  "Filtering Block " : MATLAB Function  TreatAsAtomicUnit=on
  Gain{,1..4} (5 alike) : Gain  Gain=2*pi
  MATLAB Function : MATLAB Function  TreatAsAtomicUnit=on
  MATLAB Function1 : MATLAB Function  TreatAsAtomicUnit=on
  MATLAB Function2 : MATLAB Function  TreatAsAtomicUnit=on
  MATLAB Function3 : MATLAB Function  TreatAsAtomicUnit=on
  MATLAB Function4 : MATLAB Function  TreatAsAtomicUnit=on
  Switch{,1..4} (5 alike) : Switch  Criteria=u2 ~= 0  SaturateOnIntegerOverflow=off  InputSameDT=off
  WindSpeed : Outport  VectorParamsAs1DForOutWhenUnconnected=off
  GenSpeed : Outport  Port=2  VectorParamsAs1DForOutWhenUnconnected=off
  Pitch : Outport  Port=3
  GenTorque : Outport  Port=4
  El_Power : Outport  Port=5
  wires:
  [Wind_Speed] -> Switch/3, MATLAB Function/4(u)
  MATLAB Function/1(y) -> Switch/1
  Switch/1 -> "Filtering Block "/2(wind)
  MATLAB Function1/1(y) -> Switch1/1
  Wind_Filter_Parameters/1 -> Demux/1
  Demux/2 -> Gain/1
  Demux/4 -> Gain1/1
  Switch1/1 -> "Filtering Block "/4(GenSpeed)
  Demux/3 -> [GenSpeedFilter_Switch]
  Demux/1 -> [WindSpeedFilter_Switch]
  [GenSpeedFilter_Switch] -> Switch1/2
  [WindSpeedFilter_Switch] -> Switch/2
  Demux/10 -> Gain4/1
  Gain4/1 -> MATLAB Function4/2(freq)
  "Filtering Block "/2(omega) -> GenSpeed/1
  Demux/6 -> Gain2/1
  "Filtering Block "/3(ptch) -> Pitch/1
  Demux/8 -> Gain3/1
  "Filtering Block "/4(torque) -> GenTorque/1
  "Filtering Block "/5(Power) -> El_Power/1
  "Filtering Block "/1(wnd) -> WindSpeed/1
  [Torque] -> MATLAB Function3/4(u), Switch3/3
  [Power] -> MATLAB Function4/4(u), Switch4/3
  Gain3/1 -> MATLAB Function3/2(freq)
  Power/1 -> [Power]
  Torque/1 -> [Torque]
  Pitch_in/1 -> [Pitch_In]
  Generator_speed/1 -> [Generator_Speed]
  Wind_speed/1 -> [Wind_Speed]
  SimTime/1 -> "Filtering Block "/11(time)
  [Generator_Speed] -> "Filtering Block "/3(GenSpeedNF)
  [Wind_Speed] -> "Filtering Block "/1(windNF)
  [Power] -> "Filtering Block "/10(PwrNF)
  [Pitch_In] -> "Filtering Block "/6(PitchNF)
  [Torque] -> "Filtering Block "/8(TqNF)
  Demux/5 -> [PitchFilter_Switch]
  Demux/7 -> [TorqueFilter_Switch]
  Demux/9 -> [PowerFilter_Switch]
  MATLAB Function2/1(y) -> Switch2/1
  [PitchFilter_Switch] -> Switch2/2
  Switch2/1 -> "Filtering Block "/5(Pitch)
  [TorqueFilter_Switch] -> Switch3/2
  MATLAB Function3/1(y) -> Switch3/1
  [PowerFilter_Switch] -> Switch4/2
  MATLAB Function4/1(y) -> Switch4/1
  Switch3/1 -> "Filtering Block "/7(Tq)
  Switch4/1 -> "Filtering Block "/9(Pwr)
  Demux/11 -> [LPF_ST]
  [LPF_ST] -> "Filtering Block "/12(LPF_Starting_Time)
  [Wspeed_PreWarp] -> MATLAB Function/1(w0)
  dt/1 -> [dt]
  [dt] -> MATLAB Function/3(Ts)
  [Generator_Speed] -> Switch1/3, MATLAB Function1/4(u)
  Gain1/1 -> MATLAB Function1/2(freq)
  [dt] -> MATLAB Function1/3(Ts)
  [Genspeed_PreWarp] -> MATLAB Function1/1(w0)
  [Pitch_In] -> Switch2/3, MATLAB Function2/4(u)
  Gain2/1 -> MATLAB Function2/2(freq)
  [dt] -> MATLAB Function2/3(Ts)
  [dt] -> MATLAB Function3/3(Ts)
  [dt] -> MATLAB Function4/3(Ts)
  [Pitch_PreWarp] -> MATLAB Function2/1(w0)
  Demux/12 -> [Wspeed_PreWarp]
  Demux/13 -> [Genspeed_PreWarp]
  Demux/14 -> [Pitch_PreWarp]
  Demux/15 -> [Torque_PreWarp]
  Demux/16 -> [Power_PreWarp]
  [Torque_PreWarp] -> MATLAB Function3/1(w0)
  [Power_PreWarp] -> MATLAB Function4/1(w0)
  Gain/1 -> MATLAB Function/2(freq)

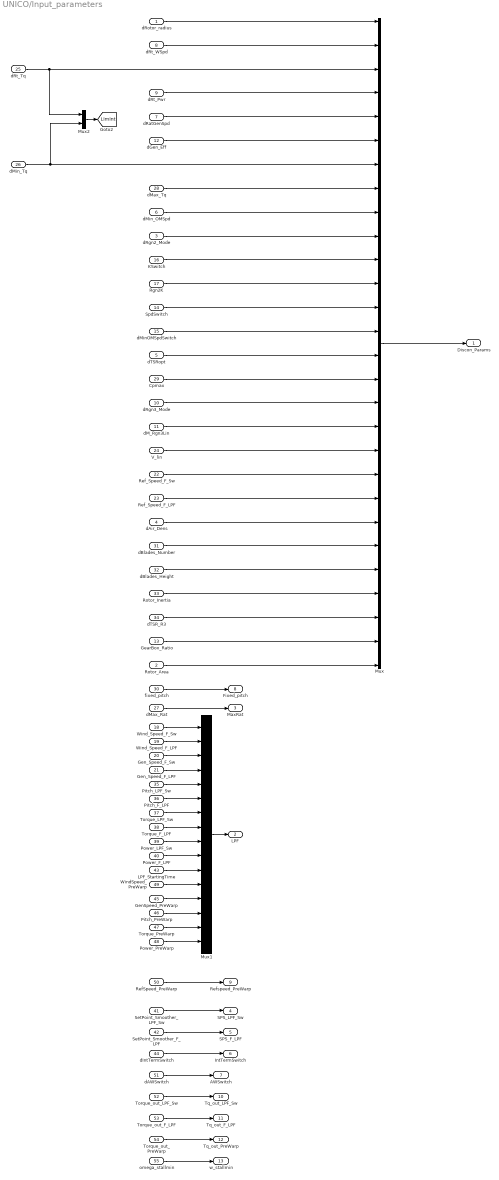
== system UNICO/Input_parameters ==
  dRotor_radius : Inport
  Rotor_Area : Inport  Port=2
  dRgn2_Mode : Inport  Port=3
  dAir_Dens : Inport  Port=4
  dTSRopt : Inport  Port=5
  dMin_OMSpd : Inport  Port=6
  dRatGenSpd : Inport  Port=7
  dRt_WSpd : Inport  Port=8
  dRt_Pwr : Inport  Port=9
  dRgn3_Mode : Inport  Port=10
  dM_Rgn3Lin : Inport  Port=11
  dGen_Eff : Inport  Port=12
  GearBox_Ratio : Inport  Port=13
  SpdSwitch : Inport  Port=14
  dMinOMSpdSwitch : Inport  Port=15
  KSwitch : Inport  Port=16
  Rgn2K : Inport  Port=17
  Wind_Speed_F_Sw : Inport  Port=18
  Wind_Speed_F_LPF : Inport  Port=19
  Gen_Speed_F_Sw : Inport  Port=20
  Gen_Speed_F_LPF : Inport  Port=21
  Ref_Speed_F_Sw : Inport  Port=22
  Ref_Speed_F_LPF : Inport  Port=23
  V_lin : Inport  Port=24
  dRt_Tq : Inport  Port=25
  dMin_Tq : Inport  Port=26
  dMax_Rat : Inport  Port=27
  dMax_Tq : Inport  Port=28
  Cpmax : Inport  Port=29
  fixed_pitch : Inport  Port=30
  dBlades_Number : Inport  Port=31
  dBlades_Height : Inport  Port=32
  Rotor_Inertia : Inport  Port=33
  dTSR_R3 : Inport  Port=34
  Pitch_LPF_Sw : Inport  Port=35
  Pitch_F_LPF : Inport  Port=36
  Torque_LPF_Sw : Inport  Port=37
  Torque_F_LPF : Inport  Port=38
  Power_LPF_Sw : Inport  Port=39
  Power_F_LPF : Inport  Port=40
  SetPoint_Smoother_LPF_Sw : Inport  Port=41
  SetPoint_Smoother_F_LPF : Inport  Port=42
  LPF_StartingTime : Inport  Port=43
  dIntTermSwitch : Inport  Port=44
  GenSpeed_PreWarp : Inport  Port=45
  Pitch_PreWarp : Inport  Port=46
  Torque_PreWarp : Inport  Port=47
  Power_PreWarp : Inport  Port=48
  WindSpeed_PreWarp : Inport  Port=49
  RefSpeed_PreWarp : Inport  Port=50
  dAWSwitch : Inport  Port=51
  Torque_out_LPF_Sw : Inport  Port=52
  Torque_out_F_LPF : Inport  Port=53
  Torque_out_PreWarp : Inport  Port=54
  omega_stallmin : Inport  Port=55
  Mux : Mux  Inputs=28
  Mux1 : Mux  Inputs=16
  Mux2 : Mux  Inputs=2
  Discon_Params : Outport
  LPF : Outport  Port=2
  MaxRat : Outport  Port=3
  SPS_LPF_Sw : Outport  Port=4
  SPS_F_LPF : Outport  Port=5
  IntTermSwitch : Outport  Port=6
  AWSwitch : Outport  Port=7
  Fixed_pitch : Outport  Port=8
  Refspeed_PreWarp : Outport  Port=9
  Tq_out_LPF_Sw : Outport  Port=10
  Tq_out_F_LPF : Outport  Port=11
  Tq_out_PreWarp : Outport  Port=12
  w_stallmin : Outport  Port=13
  tag scope: LimInt=global
  wires:
  Mux/1 -> Discon_Params/1
  dRotor_radius/1 -> Mux/1
  dRgn2_Mode/1 -> Mux/10
  dAir_Dens/1 -> Mux/22
  dTSRopt/1 -> Mux/15
  dRatGenSpd/1 -> Mux/5
  dRt_WSpd/1 -> Mux/2
  dRt_Pwr/1 -> Mux/4
  dM_Rgn3Lin/1 -> Mux/18
  dGen_Eff/1 -> Mux/6
  SpdSwitch/1 -> Mux/13
  KSwitch/1 -> Mux/11
  Rgn2K/1 -> Mux/12
  Wind_Speed_F_Sw/1 -> Mux1/1
  Wind_Speed_F_LPF/1 -> Mux1/2
  dMax_Tq/1 -> Mux/8
  dMax_Rat/1 -> MaxRat/1
  dMin_Tq/1 -> Mux/7, Mux2/2
  dRt_Tq/1 -> Mux2/1, Mux/3
  V_lin/1 -> Mux/19
  Ref_Speed_F_LPF/1 -> Mux/21
  Ref_Speed_F_Sw/1 -> Mux/20
  Gen_Speed_F_LPF/1 -> Mux1/4
  Gen_Speed_F_Sw/1 -> Mux1/3
  Mux1/1 -> LPF/1
  Mux2/1 -> [LimInt]
  dMin_OMSpd/1 -> Mux/9
  dRgn3_Mode/1 -> Mux/17
  Cpmax/1 -> Mux/16
  dMinOMSpdSwitch/1 -> Mux/14
  dBlades_Number/1 -> Mux/23
  dBlades_Height/1 -> Mux/24
  Rotor_Inertia/1 -> Mux/25
  dTSR_R3/1 -> Mux/26
  Pitch_F_LPF/1 -> Mux1/6
  Pitch_LPF_Sw/1 -> Mux1/5
  Torque_LPF_Sw/1 -> Mux1/7
  Torque_F_LPF/1 -> Mux1/8
  Power_LPF_Sw/1 -> Mux1/9
  Power_F_LPF/1 -> Mux1/10
  SetPoint_Smoother_LPF_Sw/1 -> SPS_LPF_Sw/1
  SetPoint_Smoother_F_LPF/1 -> SPS_F_LPF/1
  LPF_StartingTime/1 -> Mux1/11
  GearBox_Ratio/1 -> Mux/27
  Rotor_Area/1 -> Mux/28
  fixed_pitch/1 -> Fixed_pitch/1
  dAWSwitch/1 -> AWSwitch/1
  dIntTermSwitch/1 -> IntTermSwitch/1
  WindSpeed_PreWarp/1 -> Mux1/12
  GenSpeed_PreWarp/1 -> Mux1/13
  Pitch_PreWarp/1 -> Mux1/14
  Torque_PreWarp/1 -> Mux1/15
  Power_PreWarp/1 -> Mux1/16
  RefSpeed_PreWarp/1 -> Refspeed_PreWarp/1
  Torque_out_LPF_Sw/1 -> Tq_out_LPF_Sw/1
  Torque_out_PreWarp/1 -> Tq_out_PreWarp/1
  Torque_out_F_LPF/1 -> Tq_out_F_LPF/1
  omega_stallmin/1 -> w_stallmin/1

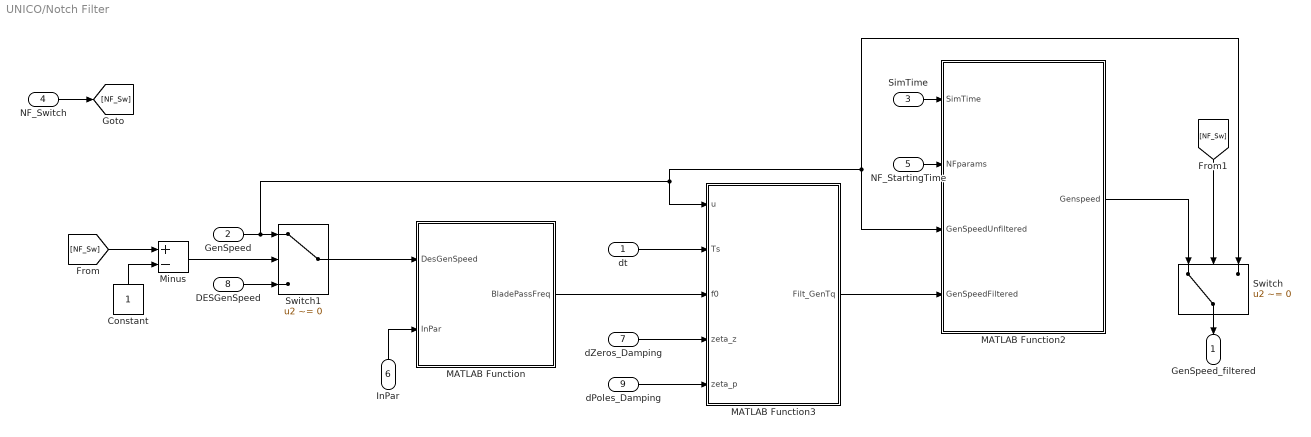
== system UNICO/Notch Filter ==
  dt : Inport
  GenSpeed : Inport  Port=2
  SimTime : Inport  Port=3
  NF_Switch : Inport  Port=4
  NF_StartingTime : Inport  Port=5
  InPar : Inport  Port=6
  dZeros_Damping : Inport  Port=7
  DESGenSpeed : Inport  Port=8
  dPoles_Damping : Inport  Port=9
  Constant : Constant
  MATLAB Function : MATLAB Function  TreatAsAtomicUnit=on
  MATLAB Function2 : MATLAB Function  TreatAsAtomicUnit=on
  MATLAB Function3 : MATLAB Function  TreatAsAtomicUnit=on
  Minus : Sum  Inputs=+-
  Switch : Switch  Criteria=u2 ~= 0  SaturateOnIntegerOverflow=off  InputSameDT=off
  Switch1 : Switch  Criteria=u2 ~= 0  SaturateOnIntegerOverflow=off  InputSameDT=off
  GenSpeed_filtered : Outport
  wires:
  dPoles_Damping/1 -> MATLAB Function3/5(zeta_p)
  dt/1 -> MATLAB Function3/2(Ts)
  dZeros_Damping/1 -> MATLAB Function3/4(zeta_z)
  MATLAB Function2/1(Genspeed) -> Switch/1
  GenSpeed/1 -> Switch/3, MATLAB Function2/3(GenSpeedUnfiltered), MATLAB Function3/1(u), Switch1/1
  MATLAB Function3/1(Filt_GenTq) -> MATLAB Function2/4(GenSpeedFiltered)
  SimTime/1 -> MATLAB Function2/1(SimTime)
  InPar/1 -> MATLAB Function/2(InPar)
  MATLAB Function/1(BladePassFreq) -> MATLAB Function3/3(f0)
  NF_StartingTime/1 -> MATLAB Function2/2(NFparams)
  Switch/1 -> GenSpeed_filtered/1
  [NF_Sw] -> Minus/1
  Constant/1 -> Minus/2
  Minus/1 -> Switch1/2
  Switch1/1 -> MATLAB Function/1(DesGenSpeed)
  DESGenSpeed/1 -> Switch1/3
  NF_Switch/1 -> [NF_Sw]
  [NF_Sw] -> Switch/2

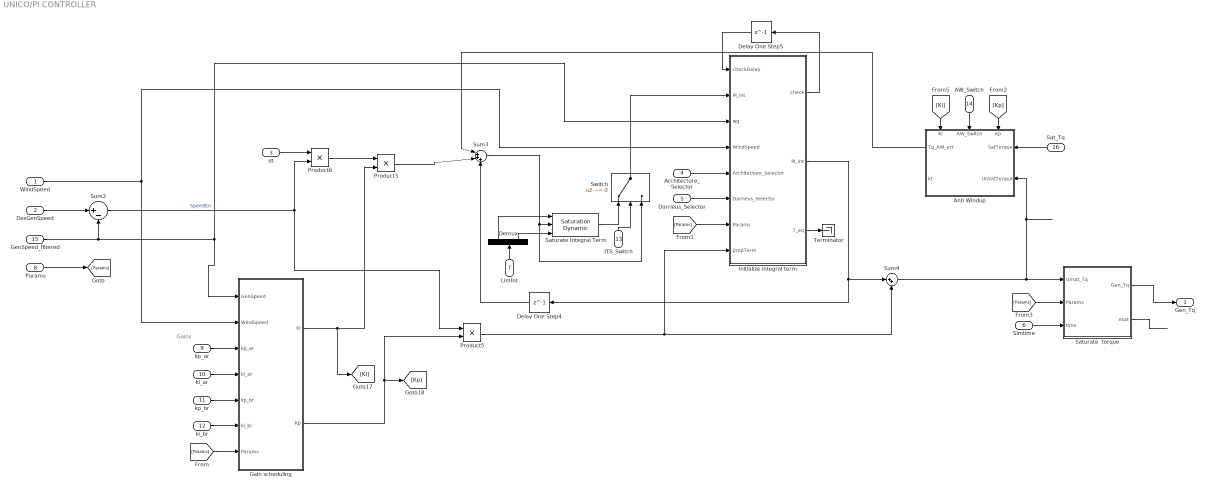
== system UNICO/PI CONTROLLER ==
  note: Gains
  WindSpeed : Inport
  DesGenSpeed : Inport  Port=2
  dt : Inport  Port=3
  Architecture_Selector : Inport  Port=4
  Darrieus_Selector : Inport  Port=5
  Simtime : Inport  Port=6
  LimInt : Inport  Port=7
  Params : Inport  Port=8
  kp_ar : Inport  Port=9
  ki_ar : Inport  Port=10
  kp_br : Inport  Port=11
  ki_br : Inport  Port=12
  ITS_Switch : Inport  Port=13
  AW_Switch : Inport  Port=14
  GenSpeed_filtered : Inport  Port=15
  Sat_Tq : Inport  Port=16
  Anti Windup : Subsystem
      settings: PortSchema="{\"entries\":[{\"content\":{\"sides\":[{\"content\":{\"connectorIds\":[\"In1\",\"In2\"]},\"type\":\"ConnectorPlacement.EquallySpacedRectSide\",\"uuid\":\"e4d44de1-1d96-4174-8cef-48dfd9e6462f\"},{\"content\":{\"connectorIds\":[\"Out1\",\"Out2\"],\"side\":\"RIGHT\"},\"type\":\"ConnectorPlacement.EquallySpacedRectSide\",\"uuid\":\"f3a799da-4ec7-4180-951d-07795f8d70de\"},{\"content\":{\"connectorIds\":[\"In3\",\"In4\",\"In5\"],\"side\":\"TOP\"},\"type\":\"ConnectorPlacement.EquallySpacedRectSide\",\"uuid\":\"9208d902-6d50-4a78-a755-8159389fc695\"}]},\"type\":\"ConnectorPlacement.EquallySpacedConnector\",\"uuid\":\"2001907f-349e-43ea-b1c8-80d5b2137fae\"}],\"packageUris\":[\"http://schema.mathworks.com/mf0/Connector/R2020b\"],\"version\":\"1.0\"}"
  Delay One Step4 : Delay  DelayLength=1
  Delay One Step5 : Delay  DelayLength=1
  Demux : Demux  Outputs=2
  Gain scheduling : MATLAB Function  TreatAsAtomicUnit=on
  Initialize integral term : MATLAB Function  TreatAsAtomicUnit=on
  Product3 : Product
  Product5 : Product
  Product6 : Product
  Saturate  torque : MATLAB Function  TreatAsAtomicUnit=on
  Saturate Integral Term : simulink/Discontinuities/Saturation Dynamic  OutMin=[]  OutMax=[]  OutDataTypeStr=Inherit: Same as second input  OutDataType=fixdt(1, 16)  OutScaling=2^-10  RndMeth=Nearest  DoSatur=off
  Sum2 : Sum  Inputs=|+-
  Sum3 : Sum  Inputs=|+++
  Sum4 : Sum  Inputs=|++
  Switch : Switch  Criteria=u2 ~= 0  SaturateOnIntegerOverflow=off  InputSameDT=off
  Terminator : Terminator
  Gen_Tq : Outport
  wires:
  Demux/1 -> Saturate Integral Term/1
  Delay One Step5/1 -> Initialize integral term/1(checkDelay)
  Product5/1 -> Sum4/2, Initialize integral term/8(propTerm)
  DesGenSpeed/1 -> Sum2/1
  Initialize integral term/1(check) -> Delay One Step5/1
  GenSpeed_filtered/1 -> Initialize integral term/3(wg), Gain scheduling/1(GenSpeed), Sum2/2
  Simtime/1 -> Saturate  torque/3(time)
  Delay One Step4/1 -> Sum3/3
  LimInt/1 -> Demux/1
  Demux/2 -> Saturate Integral Term/3
  ki_br/1 -> Gain scheduling/6(ki_br)
  Saturate  torque/1(Gen_Tq) -> Gen_Tq/1
  Sum2/1 -> Product5/1, Product6/2  "SpeedErr"
  Sum3/1 -> Switch/3, Saturate Integral Term/2
  Product6/1 -> Product3/1
  kp_ar/1 -> Gain scheduling/3(kp_ar)
  Initialize integral term/2(PI_int) -> Delay One Step4/1, Sum4/1
  WindSpeed/1 -> Initialize integral term/4(WindSpeed), Gain scheduling/2(WindSpeed)
  ki_ar/1 -> Gain scheduling/4(ki_ar)
  kp_br/1 -> Gain scheduling/5(kp_br)
  Product3/1 -> Sum3/2
  Architecture_Selector/1 -> Initialize integral term/5(Architecture_Selector)
  dt/1 -> Product6/1
  Sat_Tq/1 -> Anti Windup/1(SatTorque)
  Anti Windup/1(Tq_AW_err) -> Sum3/1
  [Ki] -> Anti Windup/5(Ki)
  [Kp] -> Anti Windup/3(Kp)
  Params/1 -> [Params]
  [Params] -> Gain scheduling/7(Params)
  [Params] -> Initialize integral term/7(Params)
  [Params] -> Saturate  torque/2(Params)
  Saturate Integral Term/1 -> Switch/1
  ITS_Switch/1 -> Switch/2
  AW_Switch/1 -> Anti Windup/4(AW_Switch)
  Darrieus_Selector/1 -> Initialize integral term/6(Darrieus_Selector)
  Switch/1 -> Initialize integral term/2("PI_int ")
  Gain scheduling/1(Ki) -> [Ki], Product3/2
  Gain scheduling/2(Kp) -> [Kp], Product5/2
  Initialize integral term/3(T_eq) -> Terminator/1
  Saturate  torque/2(esat) -> ?
  Sum4/1 -> Saturate  torque/1(Unsat_Tq), Anti Windup/2(UnSatTorque)

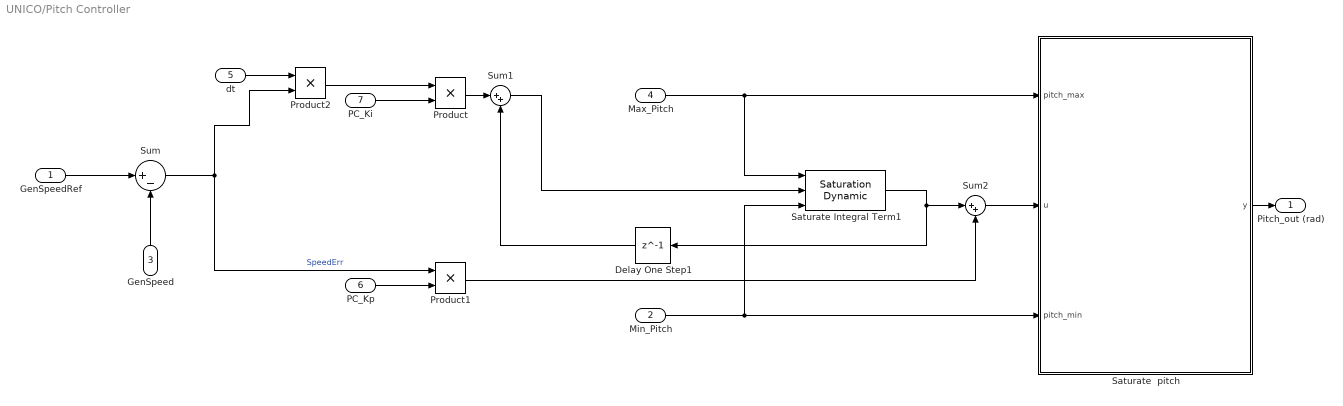
== system UNICO/Pitch Controller ==
  GenSpeedRef : Inport
  Min_Pitch : Inport  Port=2
  GenSpeed : Inport  Port=3
  Max_Pitch : Inport  Port=4
  dt : Inport  Port=5
  PC_Kp : Inport  Port=6
  PC_Ki : Inport  Port=7
  Delay One Step1 : Delay  DelayLength=1
  Product : Product
  Product1 : Product
  Product2 : Product
  Saturate  pitch : MATLAB Function  TreatAsAtomicUnit=on
  Saturate Integral Term1 : simulink/Discontinuities/Saturation Dynamic  OutMin=[]  OutMax=[]  OutDataTypeStr=Inherit: Same as second input  OutDataType=fixdt(1, 16)  OutScaling=2^-10  RndMeth=Nearest  DoSatur=off
  Sum : Sum  Inputs=|+-
  Sum1 : Sum  Inputs=|++
  Sum2 : Sum  Inputs=|++
  Pitch_out (rad) : Outport
  wires:
  GenSpeedRef/1 -> Sum/1
  Sum/1 -> Product2/2, Product1/1  "SpeedErr"
  Product/1 -> Sum1/1
  Product1/1 -> Sum2/2
  Sum1/1 -> Saturate Integral Term1/2
  dt/1 -> Product2/1
  PC_Ki/1 -> Product/2
  PC_Kp/1 -> Product1/2
  Product2/1 -> Product/1
  Delay One Step1/1 -> Sum1/2
  Saturate  pitch/1(y) -> Pitch_out (rad)/1
  Saturate Integral Term1/1 -> Delay One Step1/1, Sum2/1
  Sum2/1 -> Saturate  pitch/2(u)
  Min_Pitch/1 -> Saturate Integral Term1/3, Saturate  pitch/3(pitch_min)
  Max_Pitch/1 -> Saturate  pitch/1(pitch_max), Saturate Integral Term1/1
  GenSpeed/1 -> Sum/2

== system UNICO/Pitch Rate Limiter ==
  dt : Inport
  Pitch_Rate : Inport  Port=2
  pitch [rad] : Inport  Port=3
  Delay One Step3 : Delay  DelayLength=1
  Rate limiter : MATLAB Function  TreatAsAtomicUnit=on
  s : Outport
  wires:
  Delay One Step3/1 -> Rate limiter/1(u_b)
  Rate limiter/1(s) -> Delay One Step3/1, s/1
  dt/1 -> Rate limiter/4(dt)
  Pitch_Rate/1 -> Rate limiter/3(Pitch_Rate)
  pitch [rad]/1 -> Rate limiter/2(u)

== system UNICO/Pitch Rate Limiter1 ==
  dt : Inport
  Pitch_Rate : Inport  Port=2
  pitch [rad] : Inport  Port=3
  Delay One Step3 : Delay  DelayLength=1
  Rate limiter : MATLAB Function  TreatAsAtomicUnit=on
  s : Outport
  wires:
  Delay One Step3/1 -> Rate limiter/1(u_b)
  Rate limiter/1(s) -> Delay One Step3/1, s/1
  dt/1 -> Rate limiter/4(dt)
  Pitch_Rate/1 -> Rate limiter/3(Pitch_Rate)
  pitch [rad]/1 -> Rate limiter/2(u)

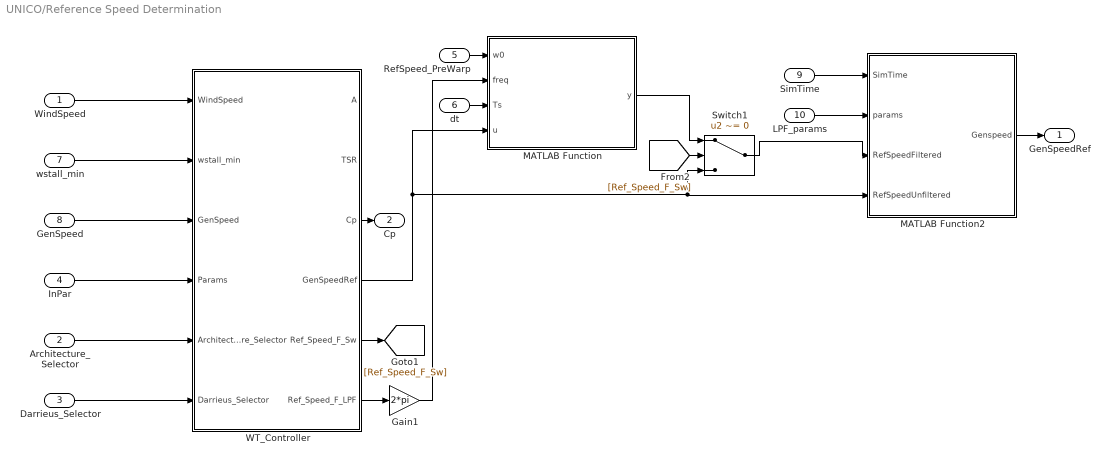
== system UNICO/Reference Speed Determination ==
  WindSpeed : Inport
  Architecture_Selector : Inport  Port=2
  Darrieus_Selector : Inport  Port=3
  InPar : Inport  Port=4
  RefSpeed_PreWarp : Inport  Port=5
  dt : Inport  Port=6
  wstall_min : Inport  Port=7
  GenSpeed : Inport  Port=8
  SimTime : Inport  Port=9
  LPF_params : Inport  Port=10
  Gain1 : Gain  Gain=2*pi
  MATLAB Function : MATLAB Function  TreatAsAtomicUnit=on
  MATLAB Function2 : MATLAB Function  TreatAsAtomicUnit=on
  Switch1 : Switch  Criteria=u2 ~= 0  SaturateOnIntegerOverflow=off  InputSameDT=off
  WT_Controller : MATLAB Function  TreatAsAtomicUnit=on
  GenSpeedRef : Outport
  Cp : Outport  Port=2
  wires:
  WindSpeed/1 -> WT_Controller/1(WindSpeed)
  WT_Controller/4(GenSpeedRef) -> MATLAB Function/4(u), Switch1/3, MATLAB Function2/4(RefSpeedUnfiltered)
  WT_Controller/6(Ref_Speed_F_LPF) -> Gain1/1
  InPar/1 -> WT_Controller/4(Params)
  GenSpeed/1 -> WT_Controller/3(GenSpeed)
  Architecture_Selector/1 -> WT_Controller/5(Architecture_Selector)
  WT_Controller/5(Ref_Speed_F_Sw) -> [Ref_Speed_F_Sw]
  [Ref_Speed_F_Sw] -> Switch1/2
  Darrieus_Selector/1 -> WT_Controller/6(Darrieus_Selector)
  MATLAB Function/1(y) -> Switch1/1
  Gain1/1 -> MATLAB Function/2(freq)
  RefSpeed_PreWarp/1 -> MATLAB Function/1(w0)
  dt/1 -> MATLAB Function/3(Ts)
  LPF_params/1 -> MATLAB Function2/2(params)
  SimTime/1 -> MATLAB Function2/1(SimTime)
  Switch1/1 -> MATLAB Function2/3(RefSpeedFiltered)
  MATLAB Function2/1(Genspeed) -> GenSpeedRef/1
  WT_Controller/3(Cp) -> Cp/1
  wstall_min/1 -> WT_Controller/2(wstall_min)
